simulink library "INP"  (R2024b)
settings: Solver=VariableStepAuto  StartTime=0.0  StopTime=10.0  RelTol=1e-3
libraries: simulink x1, INP_UNSP x1, INP_BRK x1, INP_DMP x1, INP_DRVR x1, INP_ERR x1, INP_IMU x1, INP_KEY x1, INP_SPDWHL x1, INP_SPR x1
settings Model: Creator=blatak  LastModifiedBy=jmbsp
settings ModelReferenceCC: EnableRefExpFcnMdlSchedulingChecks=on
settings RTWCC: GPUComputeCapability=3.5

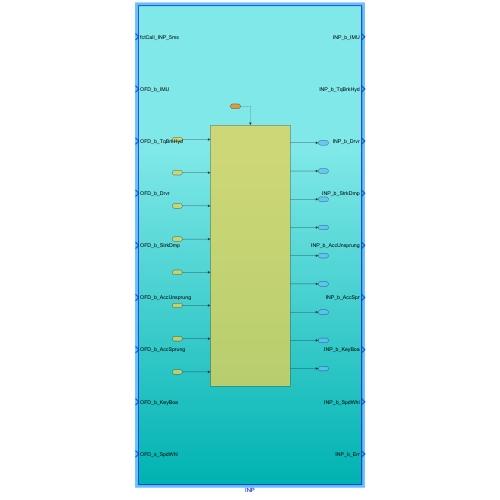
[thumbnail: Simulink's stored preview of the top-level diagram]
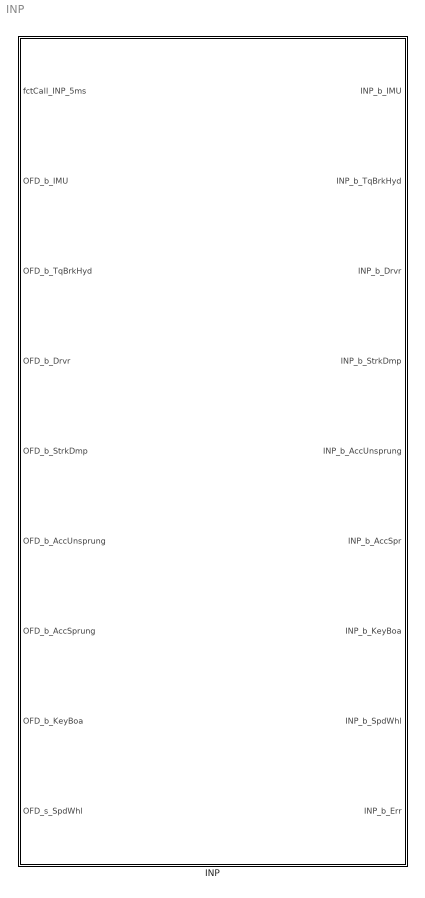
== system INP ==
  INP : Subsystem

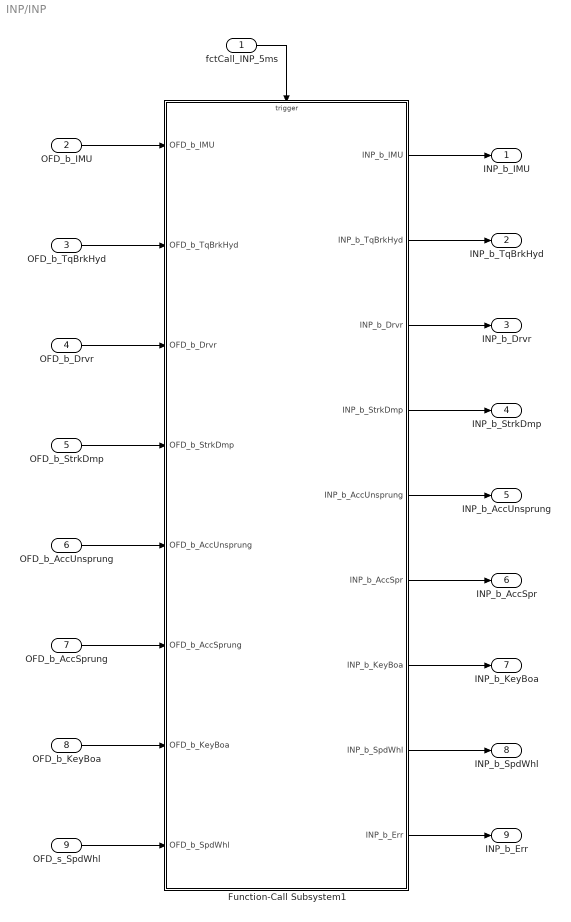
== system INP/INP ==
  fctCall_INP_5ms : Inport
  OFD_b_IMU : Inport  Port=2
  OFD_b_TqBrkHyd : Inport  Port=3
  OFD_b_Drvr : Inport  Port=4
  OFD_b_StrkDmp : Inport  Port=5
  OFD_b_AccUnsprung : Inport  Port=6
  OFD_b_AccSprung : Inport  Port=7
  OFD_b_KeyBoa : Inport  Port=8
  OFD_s_SpdWhl : Inport  Port=9
  Function-Call Subsystem1 : Subsystem  TreatAsAtomicUnit=on
  INP_b_IMU : Outport
  INP_b_TqBrkHyd : Outport  Port=2
  INP_b_Drvr : Outport  Port=3
  INP_b_StrkDmp : Outport  Port=4
  INP_b_AccUnsprung : Outport  Port=5
  INP_b_AccSpr : Outport  Port=6
  INP_b_KeyBoa : Outport  Port=7
  INP_b_SpdWhl : Outport  Port=8
  INP_b_Err : Outport  Port=9
  wires:
  Function-Call Subsystem1/7(INP_b_KeyBoa) -> INP_b_KeyBoa/1
  Function-Call Subsystem1/2(INP_b_TqBrkHyd) -> INP_b_TqBrkHyd/1
  Function-Call Subsystem1/5(INP_b_AccUnsprung) -> INP_b_AccUnsprung/1
  fctCall_INP_5ms/1 -> Function-Call Subsystem1/Trigger
  Function-Call Subsystem1/6(INP_b_AccSpr) -> INP_b_AccSpr/1
  OFD_b_Drvr/1 -> Function-Call Subsystem1/3(OFD_b_Drvr)
  Function-Call Subsystem1/3(INP_b_Drvr) -> INP_b_Drvr/1
  OFD_b_AccUnsprung/1 -> Function-Call Subsystem1/5(OFD_b_AccUnsprung)
  OFD_b_KeyBoa/1 -> Function-Call Subsystem1/7(OFD_b_KeyBoa)
  Function-Call Subsystem1/4(INP_b_StrkDmp) -> INP_b_StrkDmp/1
  OFD_b_StrkDmp/1 -> Function-Call Subsystem1/4(OFD_b_StrkDmp)
  OFD_b_TqBrkHyd/1 -> Function-Call Subsystem1/2(OFD_b_TqBrkHyd)
  OFD_b_AccSprung/1 -> Function-Call Subsystem1/6(OFD_b_AccSprung)
  Function-Call Subsystem1/1(INP_b_IMU) -> INP_b_IMU/1
  OFD_b_IMU/1 -> Function-Call Subsystem1/1(OFD_b_IMU)
  Function-Call Subsystem1/9(INP_b_Err) -> INP_b_Err/1
  OFD_s_SpdWhl/1 -> Function-Call Subsystem1/8(OFD_b_SpdWhl)
  Function-Call Subsystem1/8(INP_b_SpdWhl) -> INP_b_SpdWhl/1

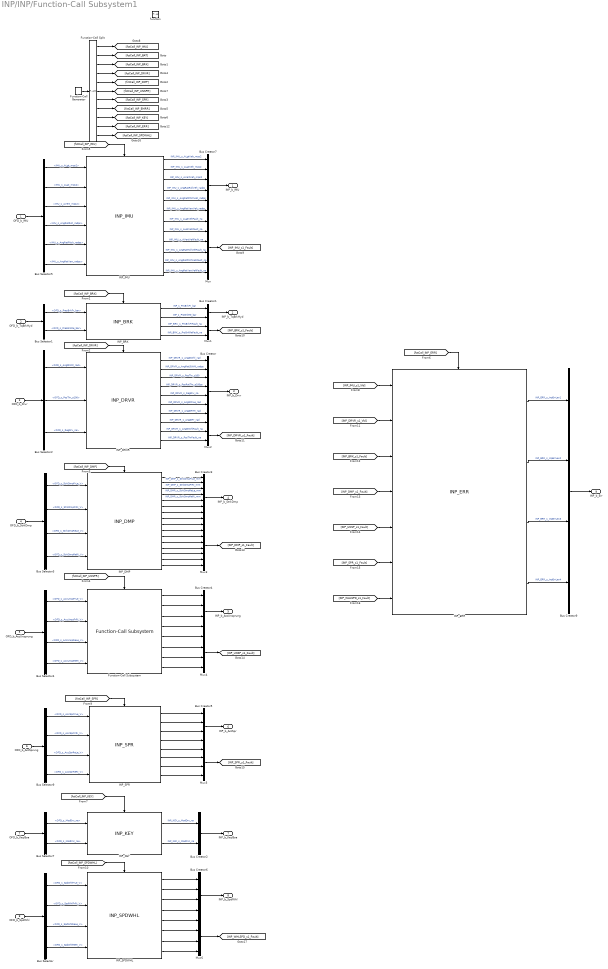
== system INP/INP/Function-Call Subsystem1 ==
  OFD_b_IMU : Inport
  OFD_b_TqBrkHyd : Inport  Port=2
  OFD_b_Drvr : Inport  Port=3
  OFD_b_StrkDmp : Inport  Port=4
  OFD_b_AccUnsprung : Inport  Port=5
  OFD_b_AccSprung : Inport  Port=6
  OFD_b_KeyBoa : Inport  Port=7
  OFD_b_SpdWhl : Inport  Port=8
  function : TriggerPort  TriggerType=function-call  VariantControl=(inherit)
  Bus Creator : BusCreator  Inputs=8  OutDataTypeStr=Bus: INP_b_Drvr
      settings: InheritFromInputs=off
  Bus Creator1 : BusCreator  Inputs=2  OutDataTypeStr=Bus: INP_b_TqBrkHyd
      settings: InheritFromInputs=off
  Bus Creator2 : BusCreator  Inputs=2  OutDataTypeStr=Bus: INP_b_KeyBoa
      settings: InheritFromInputs=off
  Bus Creator3 : BusCreator  Inputs=8  OutDataTypeStr=Bus: INP_b_StrkDmp
      settings: InheritFromInputs=off
  Bus Creator4 : BusCreator  Inputs=4  OutDataTypeStr=Bus: INP_b_AccUnsp
      settings: InheritFromInputs=off
  Bus Creator5 : BusCreator  Inputs=4  OutDataTypeStr=Bus: INP_b_AccSpr
      settings: InheritFromInputs=off
  Bus Creator6 : BusCreator  Inputs=4  OutDataTypeStr=Bus: INP_b_SpdWhl
      settings: InheritFromInputs=off
  Bus Creator7 : BusCreator  Inputs=6  OutDataTypeStr=Bus: INP_b_IMU
      settings: InheritFromInputs=off
  Bus Creator9 : BusCreator  Inputs=4  OutDataTypeStr=Bus: INP_b_Err
      settings: InheritFromInputs=off
  Bus Selector : BusSelector  OutputSignals=OFD_s_SpdWhlFrLe_V,OFD_s_SpdWhlFrRi_V,OFD_s_SpdWhlReLe_V,OFD_s_SpdWhlReRi_V
  Bus Selector1 : BusSelector  OutputSignals=OFD_s_PresBrkFr_bar,OFD_s_PresBrkRe_bar
  Bus Selector2 : BusSelector  OutputSignals=OFD_s_AngStWhl_rad,OFD_s_PosThr_p100,OFD_s_RegDrv_na
  Bus Selector3 : BusSelector  OutputSignals=OFD_s_StrkDmpFrLe_V,OFD_s_StrkDmpFrRi_V,OFD_s_StrkDmpReLe_V,OFD_s_StrkDmpReRi_V
  Bus Selector4 : BusSelector  OutputSignals=OFD_s_AccUnspFrLe_V,OFD_s_AccUnspFrRi_V,OFD_s_AccUnspReLe_V,OFD_s_AccUnspReRi_V
  Bus Selector5 : BusSelector  OutputSignals=IMU_s_ALgt_mps2,IMU_s_ALat_mps2,IMU_s_AVert_mps2,IMU_s_AngRatRoll_radps,IMU_s_AngRatPitch_radps,IMU_s_AngRatYaw_radps
  Bus Selector7 : BusSelector  OutputSignals=OFD_s_ModDrv_na,OFD_s_ModFric_na
  Bus Selector9 : BusSelector  OutputSignals=OFD_s_AccSprFrLe_V,OFD_s_AccSprFrRi_V,OFD_s_AccSprReLe_V,OFD_s_AccSprReRi_V
  Function-Call Generator : simulink/Ports & Subsystems/Function-Call Generator  sample_time=-1  numberOfIterations=1  DisallowWideOutput=off
  Function-Call Split : FunctionCallSplit  IconShape=distinctive  NumOutputPorts=11  OutputPortLayout=default
  Function-Call Subsystem : INP_UNSP/Function-Call Subsystem  SystemSampleTime=-1  VariantActivationTime=update diagram  AllowFlexibleInterface=on  Latency=0  AutoFrameSizeCalculation=off
  INP_BRK : INP_BRK/INP_BRK  SystemSampleTime=-1  VariantActivationTime=update diagram  AllowFlexibleInterface=on  Latency=0  AutoFrameSizeCalculation=off
  INP_DMP : INP_DMP/INP_DMP  SystemSampleTime=-1  VariantActivationTime=update diagram  AllowFlexibleInterface=on  Latency=0  AutoFrameSizeCalculation=off
  INP_DRVR : INP_DRVR/INP_DRVR  SystemSampleTime=-1  VariantActivationTime=update diagram  AllowFlexibleInterface=on  Latency=0  AutoFrameSizeCalculation=off
  INP_ERR : INP_ERR/INP_ERR  SystemSampleTime=-1  VariantActivationTime=update diagram  AllowFlexibleInterface=on  Latency=0  AutoFrameSizeCalculation=off
  INP_IMU : INP_IMU/INP_IMU  SystemSampleTime=-1  VariantActivationTime=update diagram  AllowFlexibleInterface=on  Latency=0  AutoFrameSizeCalculation=off
  INP_KEY : INP_KEY/INP_KEY  SystemSampleTime=-1  VariantActivationTime=update diagram  AllowFlexibleInterface=on  Latency=0  AutoFrameSizeCalculation=off
  INP_SPDWHL : INP_SPDWHL/INP_SPDWHL  SystemSampleTime=-1  VariantActivationTime=update diagram  AllowFlexibleInterface=on  Latency=0  AutoFrameSizeCalculation=off
  INP_SPR : INP_SPR/INP_SPR  SystemSampleTime=-1  VariantActivationTime=update diagram  AllowFlexibleInterface=on  Latency=0  AutoFrameSizeCalculation=off
  Mux : Mux  Inputs=6
  Mux1 : Mux  Inputs=2
  Mux2 : Mux  Inputs=2
  Mux3 : Mux  Inputs=8
  Mux4 : Mux
  Mux5 : Mux
  Mux6 : Mux
  INP_b_IMU : Outport
  INP_b_TqBrkHyd : Outport  Port=2
  INP_b_Drvr : Outport  Port=3
  INP_b_StrkDmp : Outport  Port=4
  INP_b_AccUnsprung : Outport  Port=5
  INP_b_AccSpr : Outport  Port=6
  INP_b_KeyBoa : Outport  Port=7
  INP_b_SpdWhl : Outport  Port=8
  INP_b_Err : Outport  Port=9
  wires:
  Function-Call Generator/1 -> Function-Call Split/1
  Function-Call Split/2 -> [fctCall_INP_BAT]
  Function-Call Split/3 -> [fctCall_INP_BRK]
  Function-Call Split/5 -> [fctCall_INP_DMP]
  Function-Call Split/4 -> [fctCall_INP_DRVR]
  [fctCall_INP_KEY] -> INP_KEY/Trigger
  [fctCall_INP_UNSPR] -> Function-Call Subsystem/Trigger
  [fctCall_INP_DMP] -> INP_DMP/Trigger
  [fctCall_INP_DRVR] -> INP_DRVR/Trigger
  [fctCall_INP_BRK] -> INP_BRK/Trigger
  INP_BRK/1 -> Bus Creator1/1  "INP_s_PrsBrkFr_bar"
  INP_BRK/2 -> Bus Creator1/2  "INP_s_PrsBrkRe_bar"
  Bus Creator1/1 -> INP_b_TqBrkHyd/1
  INP_DRVR/1 -> Bus Creator/1  "INP_DRVR_s_AngStWhl_rad"
  Bus Creator3/1 -> INP_b_StrkDmp/1
  Bus Creator2/1 -> INP_b_KeyBoa/1
  Bus Selector1/1 -> INP_BRK/1  "<OFD_s_PresBrkFr_bar>"
  Bus Selector1/2 -> INP_BRK/2  "<OFD_s_PresBrkRe_bar>"
  Bus Selector2/1 -> INP_DRVR/1  "<OFD_s_AngStWhl_rad>"
  Bus Selector2/2 -> INP_DRVR/2  "<OFD_s_PosThr_p100>"
  OFD_b_StrkDmp/1 -> Bus Selector3/1
  OFD_b_AccUnsprung/1 -> Bus Selector4/1
  OFD_b_KeyBoa/1 -> Bus Selector7/1
  OFD_b_Drvr/1 -> Bus Selector2/1
  OFD_b_TqBrkHyd/1 -> Bus Selector1/1
  Bus Creator4/1 -> INP_b_AccUnsprung/1
  Bus Creator/1 -> INP_b_Drvr/1
  Bus Creator5/1 -> INP_b_AccSpr/1
  OFD_b_AccSprung/1 -> Bus Selector9/1
  Function-Call Split/6 -> [fctCall_INP_UNSPR]
  Bus Selector7/1 -> INP_KEY/1  "<OFD_s_ModDrv_na>"
  Bus Selector7/2 -> INP_KEY/2  "<OFD_s_ModFric_na>"
  INP_KEY/1 -> Bus Creator2/1  "INP_KEY_s_ModDrv_na"
  INP_KEY/2 -> Bus Creator2/2  "INP_KEY_s_ModFric_na"
  Function-Call Split/8 -> [fctCall_INP_EMRR]
  Function-Call Split/7 -> [fctCall_INP_SPR]
  Function-Call Split/9 -> [fctCall_INP_KEY]
  INP_IMU/5 -> Bus Creator7/5  "INP_IMU_s_AngRatPitchVeh_radps"
  Bus Selector5/2 -> INP_IMU/2  "<IMU_s_ALat_mps2>"
  INP_IMU/1 -> Bus Creator7/1  "INP_IMU_s_ALgtVeh_mps2"
  Bus Selector5/6 -> INP_IMU/6  "<IMU_s_AngRatYaw_radps>"
  INP_IMU/3 -> Bus Creator7/3  "INP_IMU_s_AVertVeh_mps2"
  INP_IMU/4 -> Bus Creator7/4  "INP_IMU_s_AngRatRollVeh_radps"
  Bus Selector5/5 -> INP_IMU/5  "<IMU_s_AngRatPitch_radps>"
  Bus Selector5/3 -> INP_IMU/3  "<IMU_s_AVert_mps2>"
  Bus Selector5/1 -> INP_IMU/1  "<IMU_s_ALgt_mps2>"
  INP_IMU/2 -> Bus Creator7/2  "INP_IMU_s_ALatVeh_mps2"
  OFD_b_IMU/1 -> Bus Selector5/1
  INP_IMU/6 -> Bus Creator7/6  "INP_IMU_s_AngRatYawVeh_radps"
  Bus Selector5/4 -> INP_IMU/4  "<IMU_s_AngRatRoll_radps>"
  Function-Call Split/1 -> [fctCall_INP_IMU]
  [fctCall_INP_IMU] -> INP_IMU/Trigger
  INP_IMU/12 -> Mux/6  "INP_IMU_s_AngRatYawVehFault_na"
  INP_IMU/11 -> Mux/5  "INP_IMU_s_AngRatPitchVehFault_na"
  INP_IMU/10 -> Mux/4  "INP_IMU_s_AngRatRollVehFault_na"
  INP_IMU/9 -> Mux/3  "INP_IMU_s_AVertVehFault_na"
  INP_IMU/8 -> Mux/2  "INP_IMU_s_ALatVehFault_na"
  INP_IMU/7 -> Mux/1  "INP_IMU_s_ALgtVehFault_na"
  INP_BRK/3 -> Mux1/1  "INP_BRK_s_PrsBrkFrFault_na"
  INP_BRK/4 -> Mux1/2  "INP_BRK_s_PrsBrkReFault_na"
  INP_DRVR/9 -> Mux2/1  "INP_DRVR_s_AngStWhlFault_na"
  Mux/1 -> [INP_IMU_s1_Fault]
  Mux1/1 -> [INP_BRK_s1_Fault]
  Mux2/1 -> [INP_DRVR_s1_Fault]
  Function-Call Split/10 -> [fctCall_INP_ERR]
  [fctCall_INP_ERR] -> INP_ERR/Trigger
  [INP_IMU_s1_Vld] -> INP_ERR/1
  [INP_DRVR_s1_Vld] -> INP_ERR/2
  [INP_BRK_s1_Fault] -> INP_ERR/3
  INP_ERR/1 -> Bus Creator9/1  "INP_ERR_s_InpErrLev1"
  INP_ERR/2 -> Bus Creator9/2  "INP_ERR_s_InpErrLev2"
  INP_ERR/3 -> Bus Creator9/3  "INP_ERR_s_InpErrLev3"
  INP_ERR/4 -> Bus Creator9/4  "INP_ERR_s_InpErrLev4"
  Bus Creator9/1 -> INP_b_Err/1
  Bus Creator7/1 -> INP_b_IMU/1
  Bus Selector3/1 -> INP_DMP/1  "<OFD_s_StrkDmpFrLe_V>"
  Bus Selector3/2 -> INP_DMP/2  "<OFD_s_StrkDmpFrRi_V>"
  Bus Selector3/3 -> INP_DMP/3  "<OFD_s_StrkDmpReLe_V>"
  Bus Selector3/4 -> INP_DMP/4  "<OFD_s_StrkDmpReRi_V>"
  INP_DMP/1 -> Bus Creator3/1  "INP_DMP_s_StrkDmpFrLe_mm"
  INP_DMP/2 -> Bus Creator3/2  "INP_DMP_s_StrkDmpFrRi_mm"
  INP_DMP/3 -> Bus Creator3/3  "INP_DMP_s_StrkDmpReLe_mm"
  INP_DMP/4 -> Bus Creator3/4  "INP_DMP_s_StrkDmpReRi_mm"
  INP_DMP/5 -> Bus Creator3/5
  INP_DMP/6 -> Bus Creator3/6
  INP_DMP/7 -> Bus Creator3/7
  INP_DMP/8 -> Bus Creator3/8
  INP_DMP/9 -> Mux3/1
  INP_DMP/10 -> Mux3/2
  INP_DMP/11 -> Mux3/3
  INP_DMP/12 -> Mux3/4
  INP_DMP/13 -> Mux3/5
  INP_DMP/14 -> Mux3/6
  INP_DMP/15 -> Mux3/7
  INP_DMP/16 -> Mux3/8
  Mux3/1 -> [INP_DMP_s1_Fault]
  Function-Call Subsystem/1 -> Bus Creator4/1
  Function-Call Subsystem/2 -> Bus Creator4/2
  Function-Call Subsystem/3 -> Bus Creator4/3
  Function-Call Subsystem/4 -> Bus Creator4/4
  Bus Selector4/1 -> Function-Call Subsystem/1  "<OFD_s_AccUnspFrLe_V>"
  Bus Selector4/2 -> Function-Call Subsystem/2  "<OFD_s_AccUnspFrRi_V>"
  Bus Selector4/3 -> Function-Call Subsystem/3  "<OFD_s_AccUnspReLe_V>"
  Bus Selector4/4 -> Function-Call Subsystem/4  "<OFD_s_AccUnspReRi_V>"
  Function-Call Subsystem/5 -> Mux4/1
  Function-Call Subsystem/6 -> Mux4/2
  Function-Call Subsystem/7 -> Mux4/3
  Function-Call Subsystem/8 -> Mux4/4
  Mux4/1 -> [INP_UNSP_s1_Fault]
  Bus Selector9/1 -> INP_SPR/1  "<OFD_s_AccSprFrLe_V>"
  Bus Selector9/2 -> INP_SPR/2  "<OFD_s_AccSprFrRi_V>"
  Bus Selector9/3 -> INP_SPR/3  "<OFD_s_AccSprReLe_V>"
  Bus Selector9/4 -> INP_SPR/4  "<OFD_s_AccSprReRi_V>"
  INP_SPR/1 -> Bus Creator5/1
  INP_SPR/2 -> Bus Creator5/2
  INP_SPR/3 -> Bus Creator5/3
  INP_SPR/4 -> Bus Creator5/4
  INP_SPR/5 -> Mux5/1
  INP_SPR/6 -> Mux5/2
  INP_SPR/7 -> Mux5/3
  INP_SPR/8 -> Mux5/4
  Mux5/1 -> [INP_SPR_s1_Fault]
  [fctCall_INP_SPR] -> INP_SPR/Trigger
  Bus Selector2/3 -> INP_DRVR/3  "<OFD_s_RegDrv_na>"
  INP_DRVR/2 -> Bus Creator/2  "INP_DRVR_s_AngRatStWhl_radps"
  INP_DRVR/3 -> Bus Creator/3  "INP_DRVR_s_PosThr_p100"
  INP_DRVR/4 -> Bus Creator/4  "INP_DRVR_s_PosRatThr_p100ps"
  INP_DRVR/5 -> Bus Creator/5  "INP_DRVR_s_RegDrv_na"
  INP_DRVR/6 -> Bus Creator/6  "INP_DRVR_s_AngStFrLe_rad"
  INP_DRVR/7 -> Bus Creator/7  "INP_DRVR_s_AngStFrRi_rad"
  INP_DRVR/8 -> Bus Creator/8  "INP_DRVR_s_AngStFr_rad"
  INP_DRVR/10 -> Mux2/2  "INP_DRVR_s_PosThrFault_na"
  Function-Call Split/11 -> [fctCall_INP_SPDWHL]
  [fctCall_INP_SPDWHL] -> INP_SPDWHL/Trigger
  INP_SPDWHL/8 -> Mux6/4
  INP_SPDWHL/7 -> Mux6/3
  INP_SPDWHL/6 -> Mux6/2
  INP_SPDWHL/5 -> Mux6/1
  Mux6/1 -> [INP_WHLSPD_s1_Fault]
  Bus Selector/1 -> INP_SPDWHL/1  "<OFD_s_SpdWhlFrLe_V>"
  Bus Selector/2 -> INP_SPDWHL/2  "<OFD_s_SpdWhlFrRi_V>"
  Bus Selector/3 -> INP_SPDWHL/3  "<OFD_s_SpdWhlReLe_V>"
  Bus Selector/4 -> INP_SPDWHL/4  "<OFD_s_SpdWhlReRi_V>"
  OFD_b_SpdWhl/1 -> Bus Selector/1
  INP_SPDWHL/4 -> Bus Creator6/4
  INP_SPDWHL/3 -> Bus Creator6/3
  INP_SPDWHL/2 -> Bus Creator6/2
  INP_SPDWHL/1 -> Bus Creator6/1
  Bus Creator6/1 -> INP_b_SpdWhl/1
  [INP_DMP_s1_Fault] -> INP_ERR/4
  [INP_UNSP_s1_Fault] -> INP_ERR/5
  [INP_SPR_s1_Fault] -> INP_ERR/6
  [INP_WHLSPD_s1_Fault] -> INP_ERR/7
